simulink model "adders_subtractors"  (R2025b)
settings: Solver=VariableStepAuto  StartTime=0.0  StopTime=10.0  RelTol=1e-3
settings Model: Creator=Johan  LastModifiedBy=Johan

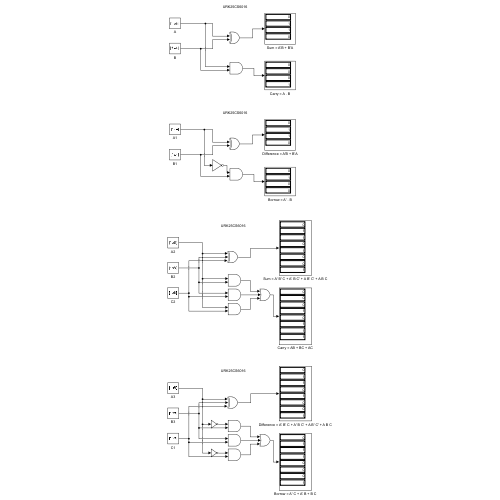
[thumbnail: Simulink's stored preview of the top-level diagram]
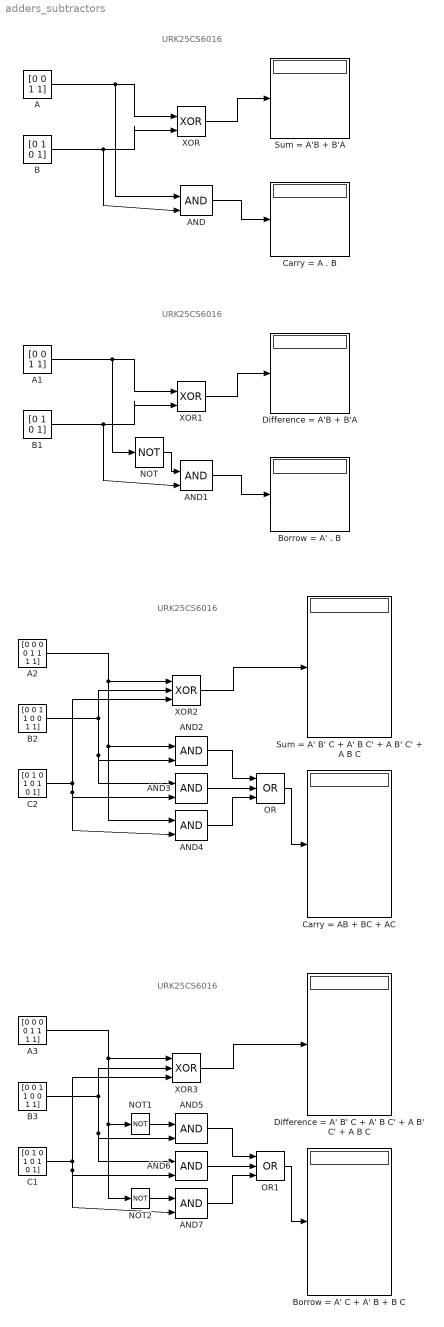
== system adders_subtractors ==
  note: URK25CS6016
  note: URK25CS6016
  note: URK25CS6016
  note: URK25CS6016
  A : Constant  Value=[0 0 1 1]
  A1 : Constant  Value=[0 0 1 1]
  A2 : Constant  Value=[0 0 0 0 1 1 1 1]
  A3 : Constant  Value=[0 0 0 0 1 1 1 1]
  AND{,1..7} (8 alike) : Logic  IconShape=distinctive  AllPortsSameDT=off  OutDataTypeStr=boolean
  B : Constant  Value=[0 1 0 1]
  B1 : Constant  Value=[0 1 0 1]
  B2 : Constant  Value=[0 0 1 1 0 0 1 1]
  B3 : Constant  Value=[0 0 1 1 0 0 1 1]
  Borrow = A' . B : Display
  Borrow = A' C + A' B + B C : Display
  C1 : Constant  Value=[0 1 0 1 0 1 0 1]
  C2 : Constant  Value=[0 1 0 1 0 1 0 1]
  Carry = A . B : Display
  Carry = AB + BC + AC : Display
  Difference = A' B' C + A' B C' + A B' C' + A B C : Display
  Difference = A'B + B'A : Display
  NOT : Logic  Operator=NOT  IconShape=distinctive  AllPortsSameDT=off  OutDataTypeStr=boolean
  NOT1 : Logic  Operator=NOT  IconShape=distinctive  AllPortsSameDT=off  OutDataTypeStr=boolean
  NOT2 : Logic  Operator=NOT  IconShape=distinctive  AllPortsSameDT=off  OutDataTypeStr=boolean
  OR : Logic  Operator=OR  Inputs=3  IconShape=distinctive  AllPortsSameDT=off  OutDataTypeStr=boolean
  OR1 : Logic  Operator=OR  Inputs=3  IconShape=distinctive  AllPortsSameDT=off  OutDataTypeStr=boolean
  Sum = A' B' C + A' B C' + A B' C' + A B C : Display
  Sum = A'B + B'A : Display
  XOR : Logic  Operator=XOR  IconShape=distinctive  AllPortsSameDT=off  OutDataTypeStr=boolean
  XOR1 : Logic  Operator=XOR  IconShape=distinctive  AllPortsSameDT=off  OutDataTypeStr=boolean
  XOR2 : Logic  Operator=XOR  Inputs=3  IconShape=distinctive  AllPortsSameDT=off  OutDataTypeStr=boolean
  XOR3 : Logic  Operator=XOR  Inputs=3  IconShape=distinctive  AllPortsSameDT=off  OutDataTypeStr=boolean
  wires:
  A/1 -> AND/1, XOR/1
  B/1 -> AND/2, XOR/2
  XOR/1 -> Sum = A'B + B'A/1
  AND/1 -> Carry = A . B/1
  AND1/1 -> Borrow = A' . B/1
  XOR1/1 -> Difference = A'B + B'A/1
  B1/1 -> XOR1/2, AND1/2
  A1/1 -> NOT/1, XOR1/1
  NOT/1 -> AND1/1
  A2/1 -> AND4/1, AND2/1, XOR2/1
  B2/1 -> AND3/1, AND2/2, XOR2/2
  XOR2/1 -> Sum = A' B' C + A' B C' + A B' C' + A B C/1
  C2/1 -> AND4/2, AND3/2, XOR2/3
  AND2/1 -> OR/1
  AND3/1 -> OR/2
  AND4/1 -> OR/3
  OR/1 -> Carry = AB + BC + AC/1
  OR1/1 -> Borrow = A' C + A' B + B C/1
  AND7/1 -> OR1/3
  AND6/1 -> OR1/2
  AND5/1 -> OR1/1
  C1/1 -> XOR3/3, AND6/2, AND7/2
  XOR3/1 -> Difference = A' B' C + A' B C' + A B' C' + A B C/1
  B3/1 -> XOR3/2, AND5/2, AND6/1
  A3/1 -> NOT2/1, NOT1/1, XOR3/1
  NOT1/1 -> AND5/1
  NOT2/1 -> AND7/1
